simulink model "Emission_Coordinator"  (R2016b)
settings: Solver=FixedStepDiscrete  StartTime=0.0  StopTime=inf  FixedStep=EmiCoorr.tiSimnTiStep_C.Value  RelTol=1e-3  EnableMultiTasking=on
undefined symbols (not defined in the file or in its folder): AuxPnmSys, PnmSys
settings Model: Creator=djuenema  LastModifiedBy=h01rauch
settings DataIOCC: SaveFormat=StructureWithTime  SaveOutput=off  DSMLogging=off  VisualizeSimOutput=off  SaveTime=off  SignalLoggingName=Results
settings OptimizationCC: BlockReduction=off  ConditionallyExecuteInputs=off  LifeSpan=inf
settings DebuggingCC: AllowSymbolicDim=off  SFUnexpectedBacktrackingDiag=warning  SFNoUnconditionalDefaultTransitionDiag=warning  SFExecutionAtInitializationDiag=none
settings ModelReferenceCC: ModelReferenceNumInstancesAllowed=Single  PropagateSignalLabelsOutOfModel=off
settings GRTTargetCC: TargetLangStandard=C89/C90 (ANSI)
settings ConfigComp: CovMetricSettings=dw  CovHtmlReporting=on  CovSaveCumulativeToWorkspaceVar=on  CovSaveSingleToWorkspaceVar=on  CovExternalEMLEnable=off

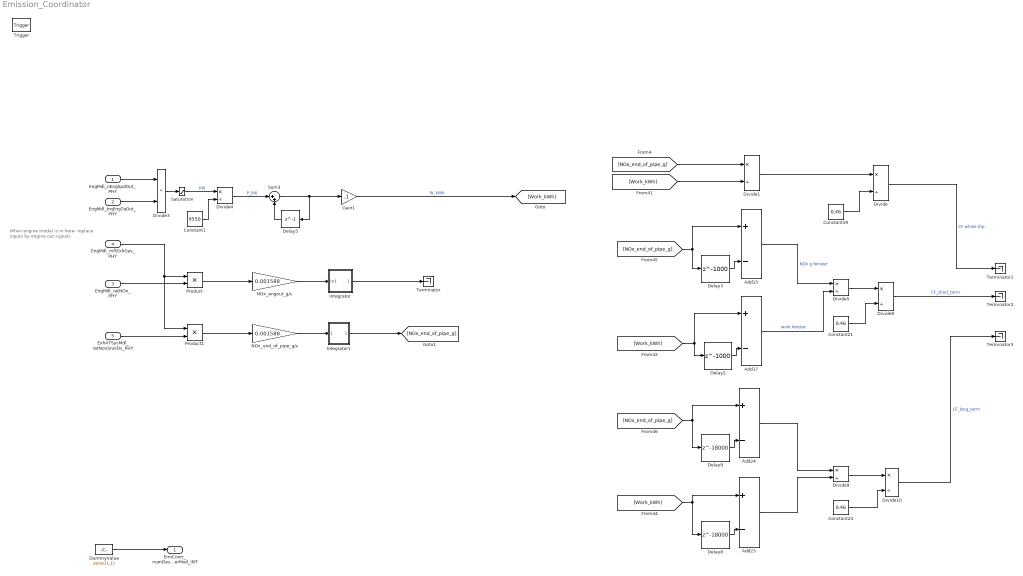
== system Emission_Coordinator ==
  note: When engine model is in here-
      | replace inputs by engine out signals
  EngMdl_nEngSpdOut_PHY : Inport
  EngMdl_trqEngTqOut_PHY : Inport  Port=2
  EngMdl_ratNOx_PHY : Inport  Port=3
  EngMdl_mflExhGas_PHY : Inport  Port=4
  ExhATSysMdl_ratNoxSnsrDs_PHY : Inport  Port=5
  Trigger : TriggerPort  TriggerType=function-call  VariantControl=Variant  PortDimensions=1
  Add{15,17,23..24} (4 alike) : Sum  Inputs=+-
  Constant1 : Constant  Value=9550
  Constant19 : Constant  Value=0.46
  Constant21 : Constant  Value=0.46
  Constant24 : Constant  Value=0.46
  Delay2 : Delay  DelayLength=1000  DelayLengthUpperLimit=AuxPnmSys.t_Dly_SigSmotng_s/PnmSys.tiSimnTiStep_C  InitialCondition=0  UseCircularBuffer=on
  Delay3 : Delay  DelayLength=1000  DelayLengthUpperLimit=AuxPnmSys.t_Dly_SigSmotng_s/PnmSys.tiSimnTiStep_C  InitialCondition=0  UseCircularBuffer=on
  Delay5 : Delay  DelayLength=1  InitialCondition=0
  Delay8 : Delay  DelayLength=18000  DelayLengthUpperLimit=AuxPnmSys.t_Dly_SigSmotng_s/PnmSys.tiSimnTiStep_C  InitialCondition=0  UseCircularBuffer=on
  Delay9 : Delay  DelayLength=18000  DelayLengthUpperLimit=AuxPnmSys.t_Dly_SigSmotng_s/PnmSys.tiSimnTiStep_C  InitialCondition=0  UseCircularBuffer=on
  Divide{,1,4..5,8..10} (7 alike) : Product  Inputs=*/
  Divide3 : Product  Inputs=**
  DummyValue : Constant  Value=zeros(1,1)  VectorParams1D=off  OutDataTypeStr=double  SampleTime=-1
  Gain1 : Gain  Gain=.1
  Integrator : Subsystem
  Integrator1 : Subsystem
  NOx_end_of_pipe_g/s : Gain  Gain=0.001588
  NOx_engout_g/s : Gain  Gain=0.001588
  Product : Product
  Product1 : Product
  Saturation : Saturate  UpperLimit=inf  LowerLimit=0
  Sum3 : Sum  Inputs=|++
  Terminator{,1..3} (4 alike) : Terminator
  EmiCoorr_numDesEngOperMod_INT : Outport
  wires:
  Gain1/1 -> [Work_kWh]  "W_kWh"
  Sum3/1 -> Gain1/1, Delay5/1
  Delay5/1 -> Sum3/2
  EngMdl_nEngSpdOut_PHY/1 -> Divide3/1
  EngMdl_trqEngTqOut_PHY/1 -> Divide3/2
  Divide3/1 -> Saturation/1
  Constant1/1 -> Divide4/2
  Divide4/1 -> Sum3/1  "P_kW"
  [NOx_end_of_pipe_g] -> Divide1/1
  Constant19/1 -> Divide/2
  Divide/1 -> Terminator1/1  "CF whole trip"
  [Work_kWh] -> Divide1/2
  Divide1/1 -> Divide/1
  Add15/1 -> Divide5/1  "NOx g fenster"
  Delay3/1 -> Add15/2
  Add17/1 -> Divide5/2  "work fenster"
  Delay2/1 -> Add17/2
  [Work_kWh] -> Add17/1, Delay2/1
  Constant21/1 -> Divide8/2
  Divide8/1 -> Terminator2/1  "CF_short_term"
  Divide5/1 -> Divide8/1
  [Work_kWh] -> Delay8/1, Add23/1
  Delay8/1 -> Add23/2
  [NOx_end_of_pipe_g] -> Delay3/1, Add15/1
  Delay9/1 -> Add24/2
  [NOx_end_of_pipe_g] -> Delay9/1, Add24/1
  Divide9/1 -> Divide10/1
  Divide10/1 -> Terminator3/1  "CF_long_term"
  Constant24/1 -> Divide10/2
  Add24/1 -> Divide9/1
  Saturation/1 -> Divide4/1  "kW"
  Add23/1 -> Divide9/2
  EngMdl_ratNOx_PHY/1 -> Product/2
  EngMdl_mflExhGas_PHY/1 -> Product1/1, Product/1
  ExhATSysMdl_ratNoxSnsrDs_PHY/1 -> Product1/2
  Product/1 -> NOx_engout_g/s/1
  Product1/1 -> NOx_end_of_pipe_g/s/1
  NOx_engout_g/s/1 -> Integrator/1(In1)
  NOx_end_of_pipe_g/s/1 -> Integrator1/1(In1)
  Integrator1/1(Out1) -> [NOx_end_of_pipe_g]
  Integrator/1(Out1) -> Terminator/1
  DummyValue/1 -> EmiCoorr_numDesEngOperMod_INT/1

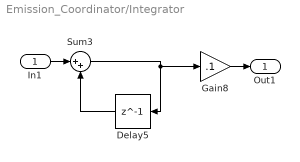
== system Emission_Coordinator/Integrator ==
  In1 : Inport
  Delay5 : Delay  DelayLength=1  InitialCondition=0
  Gain8 : Gain  Gain=.1
  Sum3 : Sum  Inputs=|++
  Out1 : Outport
  wires:
  In1/1 -> Sum3/1
  Delay5/1 -> Sum3/2
  Gain8/1 -> Out1/1
  Sum3/1 -> Gain8/1, Delay5/1

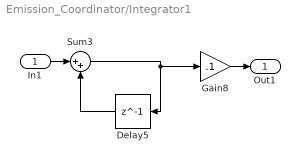
== system Emission_Coordinator/Integrator1 ==
  In1 : Inport
  Delay5 : Delay  DelayLength=1  InitialCondition=0
  Gain8 : Gain  Gain=.1
  Sum3 : Sum  Inputs=|++
  Out1 : Outport
  wires:
  Sum3/1 -> Delay5/1, Gain8/1
  Gain8/1 -> Out1/1
  Delay5/1 -> Sum3/2
  In1/1 -> Sum3/1
